simulink model "pvBatteryManagement"  (R2024b)
settings: Solver=ode1  StartTime=0.0  StopTime=10  FixedStep=5e-6  RelTol=1e-3
undefined symbols (not defined in the file): Acid, Lead
libraries: spsSeriesRLCBranchLib x8, spsVoltageMeasurementLib x5, spsCurrentMeasurementLib x4, spsIGBTDiodeLib x3, spsBatteryLib x1, spsBreakerLib x1, simulink x1, spsDiodeLib x1, slpidlib x1, spsPVArrayLib x1, spsPWMGeneratorDCDCLib x1, spsTriangleGeneratorLib x1
settings Model: Creator=Ashwin Soni  LastModifiedBy=Ashwin Soni
settings RTWCC: GPUComputeCapability=3.5

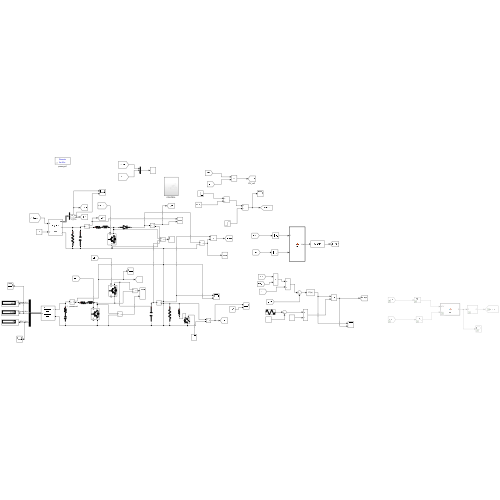
[thumbnail: Simulink's stored preview of the top-level diagram]
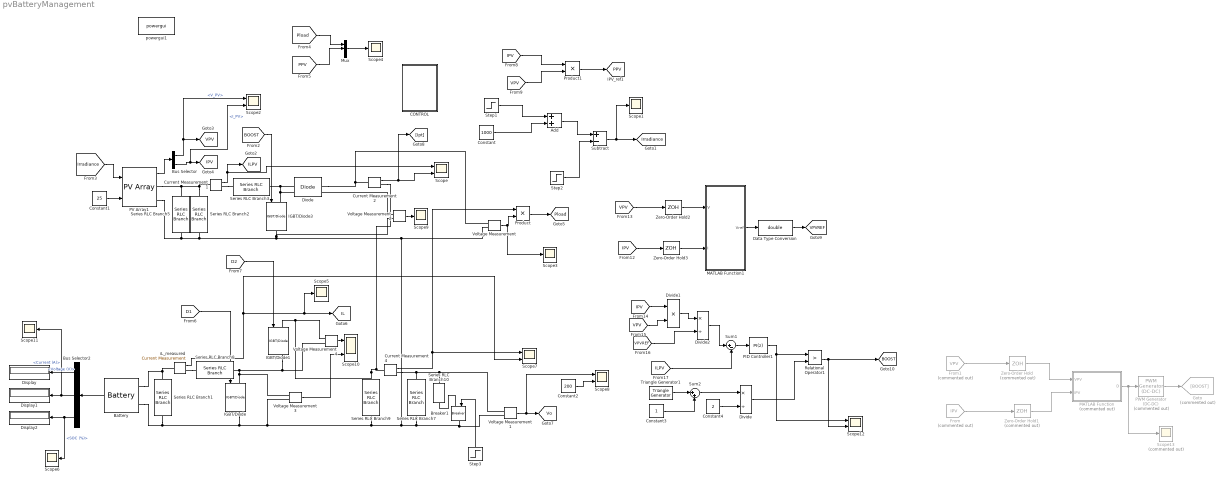
== system pvBatteryManagement ==
  Add : Sum
  Battery : spsBatteryLib/Battery  BatType=Lead-Acid  NomV=48  NomQ=26  SOC=90  Batt_Tr=30  PresetModel=on  MaxQ=27.0833  MinV=36  FullV=52.2632  Dis_rate=5.2  R=0.018462  Normal_OP=8.0672  expZone="[48.8684    0.0866667]"
  Breaker1 : spsBreakerLib/Breaker  InitialState=0  SwitchingTimes="[1/60  5/60]"  External=on  BreakerResistance=0.01  SnubberResistance=1e6  SnubberCapacitance=inf  Measurements=None  MoreParameters=on  NoBreakLoop=off
  Bus Selector : BusSelector  OutputSignals=V_PV,I_PV
  Bus Selector2 : BusSelector  OutputSignals=Voltage (V),Current (A),SOC (%)
  CONTROL : Subsystem
  Constant : Constant  Value=1000
  Constant1 : Constant  Value=25
  Constant2 : Constant  Value=200
  Constant3 : Constant
  Constant4 : Constant  Value=2
  Current Measurement1 : spsCurrentMeasurementLib/Current Measurement  PhasorSimulation=off  OutputType=Complex  PSBequivalent=0
  Current Measurement2 : spsCurrentMeasurementLib/Current Measurement  PhasorSimulation=off  OutputType=Complex  PSBequivalent=0
  Current Measurement4 : spsCurrentMeasurementLib/Current Measurement  PhasorSimulation=off  OutputType=Complex  PSBequivalent=0
  Data Type Conversion : DataTypeConversion  OutDataTypeStr=double  SaturateOnIntegerOverflow=off  RndMeth=Floor
  Diode : spsDiodeLib/Diode  Ron=0.001  Lon=0  Vf=0.8  IC=0  UseSnubber=0  Rs=inf  Cs=250e-9  Measurements=off
  Display : Display
  Display1 : Display
  Display2 : Display
  Divide : Product  Inputs=*/
  Divide1 : Product  Inputs=**
  Divide2 : Product  Inputs=*/
  From : From  Commented=on  GotoTag=IPV  TagVisibility=global
  From1 : From  Commented=on  GotoTag=VPV  TagVisibility=global
  Goto : Goto  Commented=on  GotoTag=BOOST
  IGBT/Diode : spsIGBTDiodeLib/IGBT//Diode  Ron=1e-3  Rs=1e5  Cs=inf  Measurements=on
  IGBT/Diode1 : spsIGBTDiodeLib/IGBT//Diode  Ron=1e-3  Rs=1e5  Cs=inf  Measurements=on
  IGBT/Diode3 : spsIGBTDiodeLib/IGBT//Diode  Ron=1e-3  Rs=1e5  Cs=inf  Measurements=off
  MATLAB Function : MATLAB Function  Commented=on  TreatAsAtomicUnit=on
  MATLAB Function1 : MATLAB Function  TreatAsAtomicUnit=on
  Mux : Mux  Inputs=3
  PID Controller1 : slpidlib/PID Controller  Controller=PI  Form=Parallel  TimeDomain=Discrete-time  UseExternalTs=off  SampleTime=1e-5  IntegratorMethod=Forward Euler  FilterMethod=Forward Euler  ControllerParametersSource=internal  P=5  I=1.05881  UseKiTs=off  D=0  UseExternalDerivativeSource=off  N=100  UseFilter=on  TunerSelectOption=Transfer Function Based (PID Tuner App)  InitialConditionSource=internal  InitialConditionForIntegrator=0  InitialConditionForFilter=0  DifferentiatorICPrevScaledInput=0  ExternalReset=none  TrackingMode=off  Kt=1  LimitOutput=off  SatLimitsSource=internal  UpperSaturationLimit=inf  LowerSaturationLimit=-inf  LinearizeAsGain=on  AntiWindupMode=none  Kb=1  LimitIntegrator=off  UpperIntegratorSaturationLimit=inf  LowerIntegratorSaturationLimit=-inf  POutMin=[]  POutMax=[]  IOutMin=[]  IOutMax=[]  DOutMin=[]  DOutMax=[]  NOutMin=[]  NOutMax=[]  SumOutMin=[]  SumOutMax=[]  SaturationOutMin=[]  SaturationOutMax=[]  PParamMin=[]  PParamMax=[]  IParamMin=[]  IParamMax=[]  DParamMin=[]  DParamMax=[]  NParamMin=[]  NParamMax=[]  KbParamMin=[]  KbParamMax=[]  KtParamMin=[]  KtParamMax=[]  KbOutMin=[]  KbOutMax=[]  KtOutMin=[]  KtOutMax=[]  IntegratorOutMin=[]  IntegratorOutMax=[]  FilterOutMin=[]  FilterOutMax=[]  SumI1OutMin=[]  SumI1OutMax=[]  SumI2OutMin=[]  SumI2OutMax=[]  SumI3OutMin=[]  SumI3OutMax=[]  SumI4OutMin=[]  SumI4OutMax=[]  SumDOutMin=[]  SumDOutMax=[]  DifferentiatorOutMin=[]  DifferentiatorOutMax=[]  FilterDiffOutCoefMin=[]  FilterDiffOutCoefMax=[]  ReciprocalOutMin=[]  ReciprocalOutMax=[]  SumDenOutMin=[]  SumDenOutMax=[]  SumNumOutMin=[]  SumNumOutMax=[]  DivideOutMin=[]  DivideOutMax=[]  UdiffTsProdOutMin=[]  UdiffTsProdOutMax=[]  NTsProdOutMin=[]  NTsProdOutMax=[]  UintegralTsProdOutMin=[]  UintegralTsProdOutMax=[]  UngainTsProdOutMin=[]  UngainTsProdOutMax=[]  ClampingZeroOutDataTypeStr=Inherit: Inherit via back propagation  ClampingZeroOutMin=[]  ClampingZeroOutMax=[]  FilterDenConstantOutDataTypeStr=Inherit: Inherit via back propagation  FilterDenConstantOutMin=[]  FilterDenConstantOutMax=[]  PCopyOutDataTypeStr=Inherit: Inherit via back propagation  PCopyOutMin=[]  PCopyOutMax=[]  NCopyOutDataTypeStr=Inherit: Inherit via back propagation  NCopyOutMin=[]  NCopyOutMax=[]  IntegratorContinuousStateAttributes=''  IntegratorStateMustResolveToSignalObject=off  IntegratorRTWStateStorageClass=Auto  FilterContinuousStateAttributes=''  FilterStateMustResolveToSignalObject=off  FilterRTWStateStorageClass=Auto  ParallelPVariant=InternalParameters  IdealPVariant=Disabled  IVariant=InternalParameters  DVariant=Disabled  IntegratorVariant=Discrete  SatVariant=Disabled  AWVariant=Passthrough  PCopyVariant=Disabled  TRVariant=Disabled  FdbkBlocksVariant=Forward  IdealPFdbkVariant=Disabled  SatFdbkVariant=Disabled  DerivativeFilterVariant=Disabled  NVariant=Disabled  NCopyVariant=Disabled_SignalSpec  FilterICVariant=Disabled  IntegratorICVariant=InternalICs  ExternalResetVariant=Disabled  TRSumVariant=Passthrough  SumFdbkVariant=Disabled  SumVariant=Sum_PI  TsampFilterVariant=InternalTs  TsampNgainVariant=Passthrough  TsampIntegralVariant=Disabled_SignalSpec  ExternalSaturationOutDataTypeStr=Inherit: Same as second input  DerivativeSourceVariant=Disabled  PreIntVariant=InternalPreInt
  PV Array1 : spsPVArrayLib/PV Array  Npar=2  Nser=2  PlotType=array @ 25 deg.C & specified irradiances  S_vec="[ 1000  800  600 ]"  Temp_C_vec="[ 45 25  ]"  ModuleName=Advance Solar Hydro Wind Power API-150  PlotWhenSelected=off  Pm=150.075  Ncell=72  Voc=41.8  Isc=5.05  Vm=34.5  Im=4.35  beta_Voc_pc=-0.419  alpha_Isc_pc=0.096  beta_Voc=-0.17514  alpha_Isc=0.004848  IL=5.0762  I0=1.155e-09  nI=1.0233  Rsh=71.9537  Rs=0.37337  RobustModel=off  RobustCellTemperature=313.3991  BAL=on  Tc=1e-6  Tfilter=5e-5
  PWM Generator (DC-DC) : spsPWMGeneratorDCDCLib/PWM Generator (DC-DC)  Commented=on  Fsw=10000  Ts=0
  Product : Product
  Product1 : Product
  Relational Operator1 : RelationalOperator  Operator=>  OutDataTypeStr=boolean  RndMeth=Simplest  InputSameDT=off
  Scope{,2,7..8,10,12} (6 alike) : Scope  NumInputPorts=2
  Scope{1,3..6,9,11} (7 alike) : Scope
  Scope13 : Scope  Commented=on
  Series RLC Branch1 : spsSeriesRLCBranchLib/Series RLC Branch  LConnTagsString=__new0  RConnTagsString=__new0  BranchType=RC  Resistance=0.2  Inductance=1e-3  SetiL0=off  InitialCurrent=0  Capacitance=100e-6  Setx0=off  InitialVoltage=0  Measurements=None
  Series RLC Branch10 : spsSeriesRLCBranchLib/Series RLC Branch  LConnTagsString=__new0  RConnTagsString=__new0  BranchType=R  Resistance=100  Inductance=10e-3  SetiL0=off  InitialCurrent=0  Capacitance=1e-6  Setx0=off  InitialVoltage=0  Measurements=None
  Series RLC Branch2 : spsSeriesRLCBranchLib/Series RLC Branch  LConnTagsString=__new0  RConnTagsString=__new0  BranchType=C  Resistance=1  Inductance=1e-3  SetiL0=off  InitialCurrent=0  Capacitance=1500e-6  Setx0=off  InitialVoltage=0  Measurements=None
  Series RLC Branch3 : spsSeriesRLCBranchLib/Series RLC Branch  LConnTagsString=__new0  RConnTagsString=__new0  BranchType=RL  Resistance=0.05  Inductance=13.33e-3  SetiL0=off  InitialCurrent=0  Capacitance=1e-6  Setx0=off  InitialVoltage=0  Measurements=None
  Series RLC Branch5 : spsSeriesRLCBranchLib/Series RLC Branch  LConnTagsString=__new0  RConnTagsString=__new0  BranchType=R  Resistance=10E6  Inductance=10e-3  SetiL0=off  InitialCurrent=0  Capacitance=1e-6  Setx0=off  InitialVoltage=0  Measurements=None
  Series RLC Branch7 : spsSeriesRLCBranchLib/Series RLC Branch  LConnTagsString=__new0  RConnTagsString=__new0  BranchType=R  Resistance=200  Inductance=10e-3  SetiL0=off  InitialCurrent=0  Capacitance=1e-6  Setx0=off  InitialVoltage=0  Measurements=None
  Series RLC Branch8 : spsSeriesRLCBranchLib/Series RLC Branch  LConnTagsString=__new0  RConnTagsString=__new0  BranchType=RL  Resistance=0.05  Inductance=5e-3  SetiL0=off  InitialCurrent=0  Capacitance=1e-6  Setx0=off  InitialVoltage=0  Measurements=None
  Series RLC Branch9 : spsSeriesRLCBranchLib/Series RLC Branch  LConnTagsString=__new0  RConnTagsString=__new0  BranchType=C  Resistance=1  Inductance=1e-3  SetiL0=off  InitialCurrent=0  Capacitance=220e-6  Setx0=off  InitialVoltage=0  Measurements=None
  Step1 : Step  Time=4  After=-200  SampleTime=0
  Step2 : Step  Time=6  After=200  SampleTime=0
  Step3 : Step  Time=2.5  SampleTime=0
  Subtract : Sum  Inputs=+-
  Sum1 : Sum  Inputs=|+-
  Sum2 : Sum  Inputs=|++
  Triangle Generator1 : spsTriangleGeneratorLib/Triangle Generator  Freq=10e3  Phase=90  Ts=0
  Voltage Measurement{,1..4} (5 alike) : spsVoltageMeasurementLib/Voltage Measurement  PhasorSimulation=off  OutputType=Complex  PSBequivalent=0
  Zero-Order Hold : ZeroOrderHold  Commented=on  SampleTime=1e-4
  Zero-Order Hold1 : ZeroOrderHold  Commented=on  SampleTime=1e-4
  Zero-Order Hold2 : ZeroOrderHold  SampleTime=1e-4
  Zero-Order Hold3 : ZeroOrderHold  SampleTime=1e-4
  iL_measured : spsCurrentMeasurementLib/Current Measurement  PhasorSimulation=off  OutputType=Complex  PSBequivalent=0
  powergui1 : sps_lib/powergui  Priority=1  SimulationMode=Discrete  SampleTime=5e-6  frequency=60  Iterations=50  frequencyindice=0  Pbase=100e6  ErrMax=1e-4  UnitsV=kV  UnitsW=MW  buscounter=0  FunctionMessages=off  echomessages=off  EnableUseOfTLC=off  CurrentSourceSwitches=off  DisableSnubberDevices=off  DisableRonSwitches=off  DisableVfSwitches=off  DisplayEquations=off  AutomaticDiscreteSolvers=off  SolverType=Tustin/Backward Euler (TBE)  Interpol=off  ExternalGateDelay=off  methode=off  Ts=100  x0status=blocks  SPID=on  SwTol=0  HookPort=off  NonlinearTolerance=1e-4  nMaxIteration=100  ContinueOnMaxIteration=off  RestoreLinks=warning  ResistiveCurrentMeasurement=off  Frange=[0:2:500]  Ylog=off  Xlog=on  ShowGrid=off  save=off  variable=ZData  structure=0  ZoomFFT=off  StartTime=0.0  cycles=1  DisplayStyle=1  fundamental=60  FreqAxis=off  MaxFrequency=1000  frequencyindicesteady=1  RmsSteady=1  display=off
  tag scope: BOOST=global, IL=global, ILPV=global, IPV=global, Irradiance=global, PPV=global, Pload=global, VPV=global, VPVREF=global, Vo=global
  wires:
  Voltage Measurement2/1 -> Scope9/1
  [VPV] -> Product1/2
  Mux/1 -> Scope4/1
  [IPV] -> Product1/1
  PWM Generator (DC-DC)/1 -> Goto/1
  Product1/1 -> [PPV]
  Bus Selector/1 -> Scope2/1, [VPV]  "<V_PV>"
  Current Measurement2/1 -> [Ipt], Scope/2
  [PPV] -> Mux/2
  Constant1/1 -> PV Array1/2
  Current Measurement1/1 -> Scope/1, [ILPV]
  Voltage Measurement/1 -> Scope3/1, Product/2
  PV Array1/1 -> Bus Selector/1
  MATLAB Function/1(D) -> Scope13/1, PWM Generator (DC-DC)/1
  Bus Selector/2 -> Scope2/2, [IPV]  "<I_PV>"
  [BOOST] -> IGBT/Diode3/1
  Constant/1 -> Add/2
  Add/1 -> Subtract/1
  Subtract/1 -> Scope1/1, [Irradiance]
  Product/1 -> [Pload]
  [Pload] -> Mux/1
  Step2/1 -> Subtract/2
  [Irradiance] -> PV Array1/1
  From1/1 -> Zero-Order Hold/1
  Zero-Order Hold/1 -> MATLAB Function/1(VPV)
  From/1 -> Zero-Order Hold1/1
  Zero-Order Hold1/1 -> MATLAB Function/2(IPV)
  Step3/1 -> Breaker1/1
  Voltage Measurement1/1 -> Scope8/1, [Vo]
  Bus Selector2/2 -> Scope11/1, Display1/1  "<Current (A)>"
  Voltage Measurement3/1 -> Scope10/2
  Bus Selector2/3 -> Scope6/1, Display2/1  "<SOC (%)>"
  Voltage Measurement4/1 -> Scope10/1
  Bus Selector2/1 -> Display/1  "<Voltage (V)>"
  iL_measured/1 -> Scope5/1, [IL], Scope7/2
  Current Measurement4/1 -> Product/1, Scope7/1
  [D2] -> IGBT/Diode1/1
  Battery/1 -> Bus Selector2/1
  Constant2/1 -> Scope8/2
  [D1] -> IGBT/Diode/1
  [IPV] -> Zero-Order Hold3/1
  [VPV] -> Zero-Order Hold2/1
  Data Type Conversion/1 -> [VPVREF]
  Zero-Order Hold3/1 -> MATLAB Function1/2(I)
  Zero-Order Hold2/1 -> MATLAB Function1/1(V)
  MATLAB Function1/1(Vref) -> Data Type Conversion/1
  [VPV] -> Divide1/2
  Relational Operator1/1 -> [BOOST], Scope12/2
  PID Controller1/1 -> Scope12/1, Relational Operator1/1
  Sum2/1 -> Divide/1
  Divide1/1 -> Divide2/1
  Divide2/1 -> Sum1/1
  Sum1/1 -> PID Controller1/1
  [VPVREF] -> Divide2/2
  Triangle Generator1/1 -> Sum2/1
  [IPV] -> Divide1/1
  Constant3/1 -> Sum2/2
  Divide/1 -> Relational Operator1/2
  Constant4/1 -> Divide/2
  [ILPV] -> Sum1/2
  Step1/1 -> Add/1
  connections:
  Voltage Measurement/LConn1 -- Diode/RConn1 -- Current Measurement2/LConn1
  IGBT/Diode/RConn1 -- Voltage Measurement3/LConn2 -- Series RLC Branch9/RConn1 -- Series RLC Branch7/RConn1 -- Voltage Measurement1/LConn2 -- Breaker1/RConn1 -- Voltage Measurement2/LConn2 -- IGBT/Diode3/RConn1 -- PV Array1/RConn2 -- Series RLC Branch5/RConn1 -- Series RLC Branch2/RConn1 -- Voltage Measurement/LConn2 -- Battery/LConn2 -- Series RLC Branch1/RConn1
  Series RLC Branch2/LConn1 -- Current Measurement1/LConn1 -- PV Array1/RConn1 -- Series RLC Branch5/LConn1
  Voltage Measurement2/LConn1 -- Series RLC Branch3/RConn1 -- Diode/LConn1 -- IGBT/Diode3/LConn1
  Current Measurement1/RConn1 -- Series RLC Branch3/LConn1
  IGBT/Diode1/RConn1 -- Voltage Measurement4/LConn2 -- IGBT/Diode/LConn1 -- Voltage Measurement3/LConn1 -- Series RLC Branch8/RConn1
  Current Measurement4/RConn1 -- Series RLC Branch10/LConn1 -- Voltage Measurement1/LConn1 -- Series RLC Branch7/LConn1
  Battery/LConn1 -- Series RLC Branch1/LConn1 -- iL_measured/LConn1
  Breaker1/LConn1 -- Series RLC Branch10/RConn1
  iL_measured/RConn1 -- Series RLC Branch8/LConn1
  IGBT/Diode1/LConn1 -- Current Measurement2/RConn1 -- Current Measurement4/LConn1 -- Series RLC Branch9/LConn1 -- Voltage Measurement4/LConn1

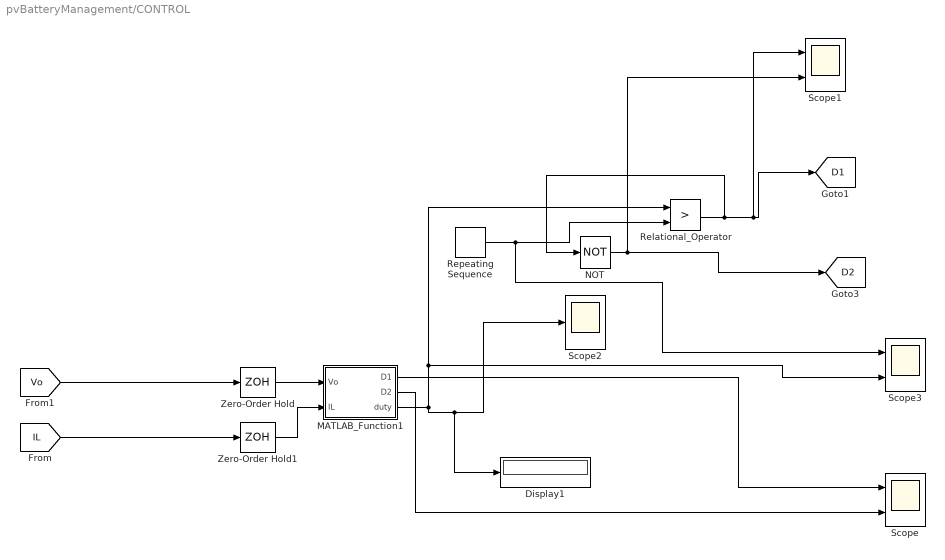
== system pvBatteryManagement/CONTROL ==
  Display1 : Display
  MATLAB_Function1 : MATLAB Function  TreatAsAtomicUnit=on
  NOT : Logic  Operator=NOT  IconShape=distinctive  AllPortsSameDT=off  OutDataTypeStr=boolean
  Relational_Operator : RelationalOperator  Operator=>  OutDataTypeStr=boolean  RndMeth=Simplest  InputSameDT=off
  Repeating Sequence : simulink/Sources/Repeating Sequence  rep_seq_t=[0 0.5 1]*(1/(10e3))  rep_seq_y=[0 1 0]
  Scope : Scope  NumInputPorts=2
  Scope1 : Scope  NumInputPorts=2
  Scope2 : Scope
  Scope3 : Scope  NumInputPorts=2
  Zero-Order Hold : ZeroOrderHold  SampleTime=1e-4
  Zero-Order Hold1 : ZeroOrderHold  SampleTime=1e-4
  tag scope: D1=global, D2=global
  wires:
  NOT/1 -> Scope1/2, [D2]
  [IL] -> Zero-Order Hold1/1
  Relational_Operator/1 -> [D1], Scope1/1, NOT/1
  Repeating Sequence/1 -> Scope3/1, Relational_Operator/2
  [Vo] -> Zero-Order Hold/1
  MATLAB_Function1/3(duty) -> Scope2/1, Display1/1, Relational_Operator/1, Scope3/2
  Zero-Order Hold/1 -> MATLAB_Function1/1(Vo)
  Zero-Order Hold1/1 -> MATLAB_Function1/2(IL)
  MATLAB_Function1/1(D1) -> Scope/1
  MATLAB_Function1/2(D2) -> Scope/2

== matlab function pvBatteryManagement/MATLAB Function1 ==
  data: V input; Vref output; I input
function Vref = fcn(V,I)

Vrefmax=200;
Vrefmin=0;
Vrefinit=200;
deltaVref=1;
persistent Vold Pold Vrefold;

if isempty(Vold)
    Vold=0;
    Pold=0;
    Vrefold=Vrefinit;
end
P=V*I;
dV=V-Vold;
dP=P-Pold;

if dP ~= 0
    if dP<0
        if dV<0
            Vref = Vrefold + deltaVref;
        else
            Vref = Vrefold - deltaVref;
        end
    else
            if dV<0
                Vref=Vrefold - deltaVref;
            else
                Vref=Vrefold + deltaVref;
            end
     end
    
else 
    Vref = Vrefold;
end
    if Vref>=Vrefmax || Vref<= Vrefmin
        Vref=Vrefold ;
    end
    Vrefold=Vref;
    Vold=V;
    Pold=P;
end

== matlab function pvBatteryManagement/MATLAB Function ==
  data: VPV input; D output; IPV input
function D = fcn(VPV,IPV)

% f = 10000hz (G)

Dinit = 0.67; %Initial value for D output
Dmax = 0.95; %Maximum value for D
Dmin = 0.1; %Minimum value for D
deltaD = 0.01; %Increment value used to increae/decrease the duty cycle D

persistent Vold Pold Dold M Iold;

dataType = 'double';

 if isempty(Vold)
     Vold=0;
     Pold=0;
     Iold=0;
     Dold=Dinit;
     M=1;
 end
 PPV = VPV*IPV;
 dVPV = VPV - Vold;
 dPPV = PPV - Pold;
 dIPV = IPV - Iold;
 M=1;
 if M <0.005
     D=Dold;
 else
     if dVPV == 0
         if dIPV == 0
             D=Dold;
         elseif dIPV>0
             D=Dold - (M*deltaD);
         else
             D=Dold + (M*deltaD);
         end
     else
         if dIPV/dVPV == -IPV/VPV
             D=Dold;
         elseif dIPV/dVPV>-IPV/VPV
             D=Dold - (M*deltaD);
         else
             D=Dold + (M*deltaD);
         end
     end
 end
 
 if D>=Dmax || D<=Dmin
     D=Dold;
 end
 
 Dold=D;
 Vold=VPV;
 Pold=PPV;
 Iold=IPV;

== matlab function pvBatteryManagement/CONTROL/MATLAB_Function1 ==
  data: D1 output; D2 output; Vo input; IL input; duty output
function [D1,D2,duty]  = control(Vo, IL)
    % Constants
    V_ref = 200;                % Reference voltage (400V)
    Kp_v = 0.09;                 % Proportional gain for voltage PI controller
    Ki_v = 40;               % Integral gain for voltage PI controller
    Kp_i = 0.02;                 % Proportional gain for current PI controller
    Ki_i = 50;              % Integral gain for current PI controller
    dead_time = 5e-6;           % Dead time in seconds (adjust as needed)
    Ts = 1e-5;                  % Sampling time in seconds

    % Persistent variables for integrators
    persistent error_v_int error_i_int;
    if isempty(error_v_int)
        error_v_int = 0;
        error_i_int = 0;
    end

    % Voltage Control Loop (Outer Loop)
    error_v = V_ref - Vo;       % Voltage error
    error_v_int = error_v_int + (error_v * Ts);  % Integrate the voltage error
    I_ref = (Kp_v * error_v) + (Ki_v * error_v_int);  % Output: Current reference
    
    % Temporary for innerloop tuning
    %I_ref = 7;

    % Current Control Loop (Inner Loop)
    error_i = I_ref - IL;       % Current error
    error_i_int = error_i_int + (error_i * Ts);  % Integrate the current error
    duty_cycle = (Kp_i * error_i) + (Ki_i * error_i_int);  % Output: Duty cycle

    duty = duty_cycle;
    
    % Clamp duty cycle to [0, 1]
    duty_cycle = max(0, min(0.95, duty_cycle));

    % Dead Time Logic
    if duty_cycle > 0.5
        D1 = duty_cycle - dead_time;   % Boost mode (Discharging battery)
        D2 = 0;                       % Disable buck mode
    else
        D1 = 0;                       % Disable boost mode
        D2 = duty_cycle - dead_time;   % Buck mode (Charging battery)
    end
    % Ensure duty cycles remain non-negative after applying dead time
    D1 = max(0, D1);
    D2 = max(0, D2);
end
